simulink subsystem "edge1x2_simple_asSubsystem"  (R2021a)
settings: Solver=VariableStepAuto  StartTime=0.0  StopTime=10.0  RelTol=1e-3
libraries: EdgesLibrary x2
settings Model: Creator=phill  LastModifiedBy=phill

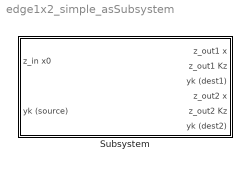
== system edge1x2_simple_asSubsystem ==
  Subsystem : Subsystem  mask{tRk=0, w1=0.5}
      mask prompts: tRk "Rk total"; w1 "weight for z_out 1"
      settings: PortSchema="{\"entries\":[{\"content\":{\"sides\":[{\"content\":{\"connectorIds\":[\"In1\",\"Out3\"]},\"type\":\"ConnectorPlacement.EquallySpacedRectSide\",\"uuid\":\"58588114-80b7-4cf3-8a8f-92af49331a70\"},{\"content\":{\"connectorIds\":[\"In2\",\"In3\",\"Out1\",\"In4\",\"In5\",\"Out2\"],\"side\":\"RIGHT\"},\"type\":\"ConnectorPlacement.EquallySpacedRectSide\",\"uuid\":\"0e7c0143-84e4-4501-996a-3b666730c0e6\"},{\"content\":{\"connectorIds\":[],\"side\":\"TOP\"},\"type\":\"ConnectorPlacement.EquallySpacedRectSide\",\"uuid\":\"990b873b-8878-4c8e-bdf4-2f621fb88a1c\"}]},\"type\":\"ConnectorPlacement.EquallySpacedConnector\",\"uuid\":\"e53b41a9-82b8-4753-89eb-fe06ea1139d8\"}],\"packageUris\":[\"http://schema.mathworks.com/mf0/Connector/R2020b\"],\"version\":\"1.0\"}"
      mask Display:
      | image('$imagefile'); % Use "Edit Image" on toolstrip to change.
      | % image('.\EdgeIconLightGrey.png');
      | disp('Simple Edge 1x2\n\n\n');
      | tRk = get_param(gcb,'tRk');
      | w1 = get_param(gcb, 'w1');
      | disp(['Rk = ', tRk, ' | w1 =  ', w1])

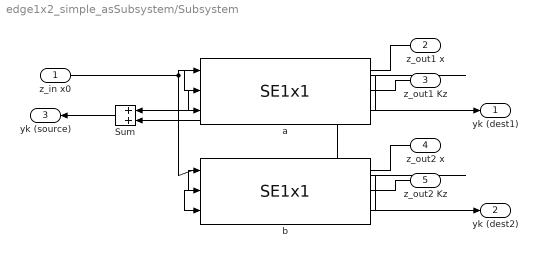
== system edge1x2_simple_asSubsystem/Subsystem ==
  z_in x0 : Inport
  z_out1 x : Inport  Port=2
  z_out1 Kz : Inport  Port=3
  z_out2 x : Inport  Port=4
  z_out2 Kz : Inport  Port=5
  Sum : Sum
  a : EdgesLibrary/SE1x1  Rk=w1*tRk
  b : EdgesLibrary/SE1x1  Rk=(1-w1)*tRk
  yk (dest1) : Outport
  yk (dest2) : Outport  Port=2
  yk (source) : Outport  Port=3
  wires:
  z_in x0/1 -> a/1, b/1
  a/1 -> yk (dest1)/1
  b/1 -> yk (dest2)/1
  Sum/1 -> yk (source)/1
  b/2 -> Sum/2
  a/2 -> Sum/1
  z_out2 x/1 -> b/2
  z_out2 Kz/1 -> b/3
  z_out1 Kz/1 -> a/3
  z_out1 x/1 -> a/2
